simulink model "gap_generation_platoon"  (R2019a)
settings: Solver=VariableStepAuto  StartTime=0.0  StopTime=25  RelTol=1e-3
values from neighbouring files (symbols this model uses):
  ehMax = 3    [sim_parameters.m]
  ehMin = -100    [sim_parameters.m]
  g0 = 1/2*maxAccel*T^2 + maxAccel*T*t1 + + 1/2*maxAccel*t1^2 + 1/6*minJerk*t1^3 -      1/(2*minAccel)*(maxAccel*T + maxAccel*t1+ 1/2*minJerk*t1^2)^2    [safeHeadway.m]    (also in sim_parameters.m = ceil(g0*10)*1.1/10)
  h = figure()    [plotKinematicsFromSimulink.m]    (also in safeHeadway.m = T + t1 -      1/minAccel*(maxAccel*T + maxAccel*t1+1/2*minJe; sim_parameters.m = ceil(h*10)*1.1/10)
  Kd = K(1)    [SimulinkScenario.m]
  Ki = K(3)    [SimulinkScenario.m]
  Kp = K(2)    [SimulinkScenario.m]
  lcStartTime = 5    [SimulinkScenario.m]
  maxAcc = 4    [sim_parameters.m]
  maxJerk = 40    [sim_parameters.m]
  minAcc = -8    [sim_parameters.m]
  minJerk = -75    [sim_parameters.m]
  p = 10    [sim_parameters.m]
  vehMass = 2000    [sim_parameters.m]
  velKi = KiVelControl    [SimulinkScenario.m]
  vLen = lf+lr    (= 3)    [sim_parameters.m]
libraries: autolibshared x5
settings Model: Creator=fvall  LastModifiedBy=fvall

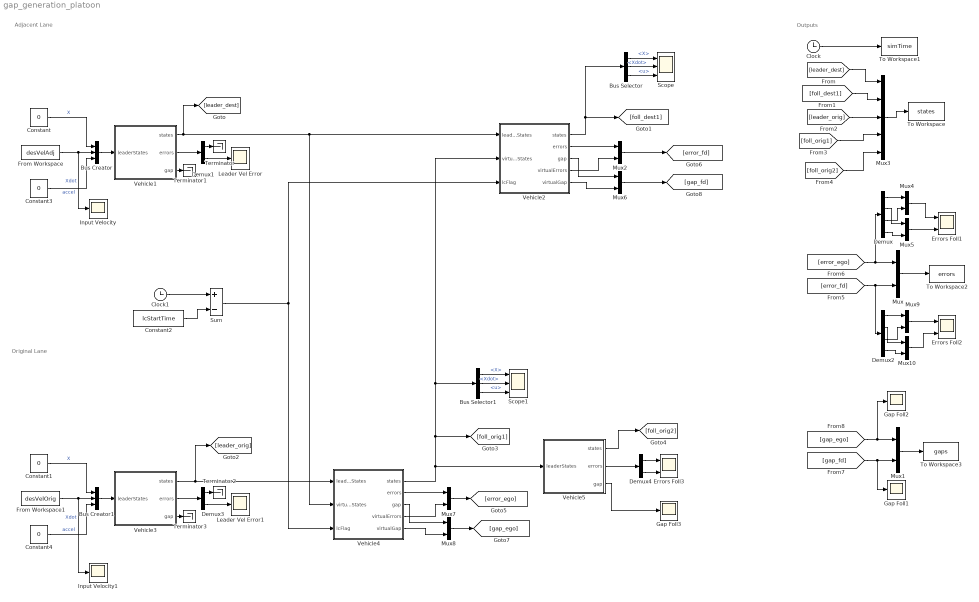
== system gap_generation_platoon ==
  note: Original Lane
  note: Adjacent Lane
  note: Outputs
  Bus Creator : BusCreator  Inputs=3
  Bus Creator1 : BusCreator  Inputs=3
  Bus Selector : BusSelector  OutputSignals=X,Xdot,u
  Bus Selector1 : BusSelector  OutputSignals=X,Xdot,u
  Clock : Clock
  Clock1 : Clock
  Constant{,1,3..4} (4 alike) : Constant  Value=0
  Constant2 : Constant  Value=lcStartTime
  Demux : Demux
  Demux1 : Demux  Outputs=2
  Demux2 : Demux
  Demux3 : Demux  Outputs=2
  Demux4 : Demux  Outputs=2
  Errors Foll1 : Scope  NumInputPorts=2
  Errors Foll2 : Scope  NumInputPorts=2
  Errors Foll3 : Scope  NumInputPorts=2
  From Workspace : FromWorkspace  VariableName=desVelAdj  SampleTime=0
  From Workspace1 : FromWorkspace  VariableName=desVelOrig  SampleTime=0
  Gap Foll1 : Scope
  Gap Foll2 : Scope
  Gap Foll3 : Scope
  Input Velocity : Scope
  Input Velocity1 : Scope
  Leader Vel Error : Scope
  Leader Vel Error1 : Scope
  Mux{,1..2,4..10} (10 alike) : Mux  Inputs=2
  Mux3 : Mux  Inputs=5
  Scope : Scope  NumInputPorts=3
  Scope1 : Scope  NumInputPorts=3
  Sum : Sum  Inputs=+-
  Terminator{,1..3} (4 alike) : Terminator
  To Workspace : ToWorkspace  VariableName=states  SampleTime=-1
  To Workspace1 : ToWorkspace  VariableName=simTime  SampleTime=-1
  To Workspace2 : ToWorkspace  VariableName=errors  SampleTime=-1
  To Workspace3 : ToWorkspace  VariableName=gaps  SampleTime=-1
  Vehicle1 : Subsystem  mask{m=vehMass, lf=vLen/2, lr=vLen/2, maxAcceleration=maxAcc, minAcceleration=minAcc, maxJerk=maxJerk, minJerk=minJerk, X_o=9.71, initVel=20, Y_o=3.6, h=h, g0=g0, minHeadwayError=ehMin, maxHeadwayError=ehMax, velFilterGain=p, Kd=Kd, Kp=Kp, Ki=Ki, VelKi=velKi}
      mask prompts: m "autoblks_shared:autoblkVehBody3DofLat:blkPrm_m"; lf "autoblks_shared:autoblkVehBody3DofLat:blkPrm_a"; lr "autoblks_shared:autoblkVehBody3DofLat:blkPrm_b"; maxAcceleration "Max Acceleration"; minAcceleration "Min Acceleration"; maxJerk "Max Jerk"; minJerk "Min Jerk"; X_o "autoblks_shared:autoblkVehBody3DofLat:blkPrm_X_o"; initVel "autoblks_shared:autoblkVehBody3DofLat:blkPrm_xdot_o"; Y_o "autoblks_shared:autoblkVehBody3DofLat:blkPrm_Y_o"; h "Time Headway"; g0 "Standstill Gap"; minHeadwayError "Min Headway Error"; maxHeadwayError "Max Headway Error"; velFilterGain "Velocity Filter Gain"
      mask TypeOptions m: Vehicle Body 3DOF Single Track/m
      mask TypeOptions lf: Vehicle Body 3DOF Single Track/a
      mask TypeOptions lr: Vehicle Body 3DOF Single Track/b
      mask TypeOptions X_o: Vehicle Body 3DOF Single Track/X_o
      mask TypeOptions initVel: Vehicle Body 3DOF Single Track/xdot_o
      mask TypeOptions Y_o: Vehicle Body 3DOF Single Track/Y_o
      mask TypeOptions Kd: ACC/Kd/Gain
      mask TypeOptions Kp: ACC/Kp/Gain
      mask TypeOptions Ki: ACC/Ki/Gain
      mask TypeOptions VelKi: ACC/VelKi/Gain
      mask DialogControl DescGroupVar Prompt: 3DOF Vehicle with ACC
      mask DialogControl DescTextVar Prompt: Vehicle with ACC. The vehicle model is Simulink's 3DOF single track vehicle body. The controller is a PID with constant headway including headway error saturation and filtered leader velocity.
      mask DialogControl ParameterGroupVar Prompt: Vehicle Parameters
      mask DialogControl m Prompt: Vehicle mass, m [kg]:
      mask DialogControl lf Prompt: Longitudinal distance from center of mass to front axle, a [m]:
      mask DialogControl lr Prompt: Longitudinal distance from center of mass to rear axle, b [m]:
      mask DialogControl X_o Prompt: Initial inertial frame longitudinal position, X_o [m]:
      mask DialogControl initVel Prompt: Initial longitudinal velocity, xdot_o [m/s]:
      mask DialogControl Y_o Prompt: Initial inertial frame lateral displacement, Y_o [m]:
      mask DialogControl Container3 Prompt: Controller Parameters
  Vehicle2 : Subsystem  mask{m=vehMass, lf=vLen/2, lr=vLen/2, maxAcceleration=maxAcc, minAcceleration=minAcc, maxJerk=maxJerk, minJerk=minJerk, X_o=0, initVel=20, Y_o=3.6, h=h, g0=g0, minHeadwayError=ehMin, maxHeadwayError=ehMax, velFilterGain=p, Kd=Kd, Kp=Kp, Ki=Ki, VelKi=velKi}
      mask prompts: m "autoblks_shared:autoblkVehBody3DofLat:blkPrm_m"; lf "autoblks_shared:autoblkVehBody3DofLat:blkPrm_a"; lr "autoblks_shared:autoblkVehBody3DofLat:blkPrm_b"; maxAcceleration "Max Acceleration"; minAcceleration "Min Acceleration"; maxJerk "Max Jerk"; minJerk "Min Jerk"; X_o "autoblks_shared:autoblkVehBody3DofLat:blkPrm_X_o"; initVel "autoblks_shared:autoblkVehBody3DofLat:blkPrm_xdot_o"; Y_o "autoblks_shared:autoblkVehBody3DofLat:blkPrm_Y_o"; h "Time Headway"; g0 "Standstill Gap"; minHeadwayError "Min Headway Error"; maxHeadwayError "Max Headway Error"; velFilterGain "Velocity Filter Gain"
      mask TypeOptions m: Vehicle Body 3DOF Single Track/m
      mask TypeOptions lf: Vehicle Body 3DOF Single Track/a
      mask TypeOptions lr: Vehicle Body 3DOF Single Track/b
      mask TypeOptions X_o: Vehicle Body 3DOF Single Track/X_o
      mask TypeOptions initVel: Vehicle Body 3DOF Single Track/xdot_o
      mask TypeOptions Y_o: Vehicle Body 3DOF Single Track/Y_o
      mask TypeOptions Kd: ACC/Kd/Gain
      mask TypeOptions Kp: ACC/Kp/Gain
      mask TypeOptions Ki: ACC/Ki/Gain
      mask TypeOptions VelKi: ACC/VelKi/Gain
      mask DialogControl DescGroupVar Prompt: 3DOF Vehicle with ACC
      mask DialogControl DescTextVar Prompt: Vehicle with ACC. The vehicle model is Simulink's 3DOF single track vehicle body. The controller is a PID with constant headway including headway error saturation and filtered leader velocity.
      mask DialogControl ParameterGroupVar Prompt: Vehicle Parameters
      mask DialogControl m Prompt: Vehicle mass, m [kg]:
      mask DialogControl lf Prompt: Longitudinal distance from center of mass to front axle, a [m]:
      mask DialogControl lr Prompt: Longitudinal distance from center of mass to rear axle, b [m]:
      mask DialogControl X_o Prompt: Initial inertial frame longitudinal position, X_o [m]:
      mask DialogControl initVel Prompt: Initial longitudinal velocity, xdot_o [m/s]:
      mask DialogControl Y_o Prompt: Initial inertial frame lateral displacement, Y_o [m]:
      mask DialogControl Container3 Prompt: Controller Parameters
  Vehicle3 : Subsystem  mask{m=vehMass, lf=vLen/2, lr=vLen/2, maxAcceleration=maxAcc, minAcceleration=minAcc, maxJerk=maxJerk, minJerk=minJerk, X_o=19.42, initVel=20, Y_o=0, h=h, g0=g0, minHeadwayError=ehMin, maxHeadwayError=ehMax, velFilterGain=p, Kd=Kd, Kp=Kp, Ki=Ki, VelKi=velKi}
      mask prompts: m "autoblks_shared:autoblkVehBody3DofLat:blkPrm_m"; lf "autoblks_shared:autoblkVehBody3DofLat:blkPrm_a"; lr "autoblks_shared:autoblkVehBody3DofLat:blkPrm_b"; maxAcceleration "Max Acceleration"; minAcceleration "Min Acceleration"; maxJerk "Max Jerk"; minJerk "Min Jerk"; X_o "autoblks_shared:autoblkVehBody3DofLat:blkPrm_X_o"; initVel "autoblks_shared:autoblkVehBody3DofLat:blkPrm_xdot_o"; Y_o "autoblks_shared:autoblkVehBody3DofLat:blkPrm_Y_o"; h "Time Headway"; g0 "Standstill Gap"; minHeadwayError "Min Headway Error"; maxHeadwayError "Max Headway Error"; velFilterGain "Velocity Filter Gain"
      mask TypeOptions m: Vehicle Body 3DOF Single Track/m
      mask TypeOptions lf: Vehicle Body 3DOF Single Track/a
      mask TypeOptions lr: Vehicle Body 3DOF Single Track/b
      mask TypeOptions X_o: Vehicle Body 3DOF Single Track/X_o
      mask TypeOptions initVel: Vehicle Body 3DOF Single Track/xdot_o
      mask TypeOptions Y_o: Vehicle Body 3DOF Single Track/Y_o
      mask TypeOptions Kd: ACC/Kd/Gain
      mask TypeOptions Kp: ACC/Kp/Gain
      mask TypeOptions Ki: ACC/Ki/Gain
      mask TypeOptions VelKi: ACC/VelKi/Gain
      mask DialogControl DescGroupVar Prompt: 3DOF Vehicle with ACC
      mask DialogControl DescTextVar Prompt: Vehicle with ACC. The vehicle model is Simulink's 3DOF single track vehicle body. The controller is a PID with constant headway including headway error saturation and filtered leader velocity.
      mask DialogControl ParameterGroupVar Prompt: Vehicle Parameters
      mask DialogControl m Prompt: Vehicle mass, m [kg]:
      mask DialogControl lf Prompt: Longitudinal distance from center of mass to front axle, a [m]:
      mask DialogControl lr Prompt: Longitudinal distance from center of mass to rear axle, b [m]:
      mask DialogControl X_o Prompt: Initial inertial frame longitudinal position, X_o [m]:
      mask DialogControl initVel Prompt: Initial longitudinal velocity, xdot_o [m/s]:
      mask DialogControl Y_o Prompt: Initial inertial frame lateral displacement, Y_o [m]:
      mask DialogControl Container3 Prompt: Controller Parameters
  Vehicle4 : Subsystem  mask{m=vehMass, lf=vLen/2, lr=vLen/2, maxAcceleration=maxAcc, minAcceleration=minAcc, maxJerk=maxJerk, minJerk=minJerk, X_o=9.71, initVel=20, Y_o=0, h=h, g0=g0, minHeadwayError=ehMin, maxHeadwayError=ehMax, velFilterGain=p, Kd=Kd, Kp=Kp, Ki=Ki, VelKi=velKi}
      mask prompts: m "autoblks_shared:autoblkVehBody3DofLat:blkPrm_m"; lf "autoblks_shared:autoblkVehBody3DofLat:blkPrm_a"; lr "autoblks_shared:autoblkVehBody3DofLat:blkPrm_b"; maxAcceleration "Max Acceleration"; minAcceleration "Min Acceleration"; maxJerk "Max Jerk"; minJerk "Min Jerk"; X_o "autoblks_shared:autoblkVehBody3DofLat:blkPrm_X_o"; initVel "autoblks_shared:autoblkVehBody3DofLat:blkPrm_xdot_o"; Y_o "autoblks_shared:autoblkVehBody3DofLat:blkPrm_Y_o"; h "Time Headway"; g0 "Standstill Gap"; minHeadwayError "Min Headway Error"; maxHeadwayError "Max Headway Error"; velFilterGain "Velocity Filter Gain"
      mask TypeOptions m: Vehicle Body 3DOF Single Track/m
      mask TypeOptions lf: Vehicle Body 3DOF Single Track/a
      mask TypeOptions lr: Vehicle Body 3DOF Single Track/b
      mask TypeOptions X_o: Vehicle Body 3DOF Single Track/X_o
      mask TypeOptions initVel: Vehicle Body 3DOF Single Track/xdot_o
      mask TypeOptions Y_o: Vehicle Body 3DOF Single Track/Y_o
      mask TypeOptions Kd: ACC/Kd/Gain
      mask TypeOptions Kp: ACC/Kp/Gain
      mask TypeOptions Ki: ACC/Ki/Gain
      mask TypeOptions VelKi: ACC/VelKi/Gain
      mask DialogControl DescGroupVar Prompt: 3DOF Vehicle with ACC
      mask DialogControl DescTextVar Prompt: Vehicle with ACC. The vehicle model is Simulink's 3DOF single track vehicle body. The controller is a PID with constant headway including headway error saturation and filtered leader velocity.
      mask DialogControl ParameterGroupVar Prompt: Vehicle Parameters
      mask DialogControl m Prompt: Vehicle mass, m [kg]:
      mask DialogControl lf Prompt: Longitudinal distance from center of mass to front axle, a [m]:
      mask DialogControl lr Prompt: Longitudinal distance from center of mass to rear axle, b [m]:
      mask DialogControl X_o Prompt: Initial inertial frame longitudinal position, X_o [m]:
      mask DialogControl initVel Prompt: Initial longitudinal velocity, xdot_o [m/s]:
      mask DialogControl Y_o Prompt: Initial inertial frame lateral displacement, Y_o [m]:
      mask DialogControl Container3 Prompt: Controller Parameters
  Vehicle5 : Subsystem  mask{m=vehMass, lf=vLen/2, lr=vLen/2, maxAcceleration=maxAcc, minAcceleration=minAcc, maxJerk=maxJerk, minJerk=minJerk, X_o=0, initVel=20, Y_o=0, h=h, g0=g0, minHeadwayError=ehMin, maxHeadwayError=ehMax, velFilterGain=p, Kd=Kd, Kp=Kp, Ki=Ki, VelKi=velKi}
      mask prompts: m "autoblks_shared:autoblkVehBody3DofLat:blkPrm_m"; lf "autoblks_shared:autoblkVehBody3DofLat:blkPrm_a"; lr "autoblks_shared:autoblkVehBody3DofLat:blkPrm_b"; maxAcceleration "Max Acceleration"; minAcceleration "Min Acceleration"; maxJerk "Max Jerk"; minJerk "Min Jerk"; X_o "autoblks_shared:autoblkVehBody3DofLat:blkPrm_X_o"; initVel "autoblks_shared:autoblkVehBody3DofLat:blkPrm_xdot_o"; Y_o "autoblks_shared:autoblkVehBody3DofLat:blkPrm_Y_o"; h "Time Headway"; g0 "Standstill Gap"; minHeadwayError "Min Headway Error"; maxHeadwayError "Max Headway Error"; velFilterGain "Velocity Filter Gain"
      mask TypeOptions m: Vehicle Body 3DOF Single Track/m
      mask TypeOptions lf: Vehicle Body 3DOF Single Track/a
      mask TypeOptions lr: Vehicle Body 3DOF Single Track/b
      mask TypeOptions X_o: Vehicle Body 3DOF Single Track/X_o
      mask TypeOptions initVel: Vehicle Body 3DOF Single Track/xdot_o
      mask TypeOptions Y_o: Vehicle Body 3DOF Single Track/Y_o
      mask TypeOptions Kd: ACC/Kd/Gain
      mask TypeOptions Kp: ACC/Kp/Gain
      mask TypeOptions Ki: ACC/Ki/Gain
      mask TypeOptions VelKi: ACC/VelKi/Gain
      mask DialogControl DescGroupVar Prompt: 3DOF Vehicle with ACC
      mask DialogControl DescTextVar Prompt: Vehicle with ACC. The vehicle model is Simulink's 3DOF single track vehicle body. The controller is a PID with constant headway including headway error saturation and filtered leader velocity.
      mask DialogControl ParameterGroupVar Prompt: Vehicle Parameters
      mask DialogControl m Prompt: Vehicle mass, m [kg]:
      mask DialogControl lf Prompt: Longitudinal distance from center of mass to front axle, a [m]:
      mask DialogControl lr Prompt: Longitudinal distance from center of mass to rear axle, b [m]:
      mask DialogControl X_o Prompt: Initial inertial frame longitudinal position, X_o [m]:
      mask DialogControl initVel Prompt: Initial longitudinal velocity, xdot_o [m/s]:
      mask DialogControl Y_o Prompt: Initial inertial frame lateral displacement, Y_o [m]:
      mask DialogControl Container3 Prompt: Controller Parameters
  wires:
  Vehicle2/1(states) -> Bus Selector/1, [foll_dest1]
  Demux1/1 -> Terminator/1
  Demux1/2 -> Leader Vel Error/1
  Vehicle1/3(gap) -> Terminator1/1
  From Workspace/1 -> Bus Creator/2, Input Velocity/1  "Xdot"
  Vehicle1/2(errors) -> Demux1/1
  Clock/1 -> To Workspace1/1
  [foll_dest1] -> Mux3/2
  [leader_dest] -> Mux3/1
  Mux3/1 -> To Workspace/1
  Demux3/2 -> Leader Vel Error1/1
  Demux3/1 -> Terminator2/1
  Vehicle4/1(states) -> Vehicle5/1(leaderStates), Bus Selector1/1, Vehicle2/2(virtualLeaderStates), [foll_orig1]
  Vehicle3/1(states) -> [leader_orig], Vehicle4/1(leaderStates)
  Vehicle3/3(gap) -> Terminator3/1
  [leader_orig] -> Mux3/3
  [foll_orig1] -> Mux3/4
  Vehicle5/3(gap) -> Gap Foll3/1
  Vehicle5/2(errors) -> Demux4/1
  Demux4/1 -> Errors Foll3/1
  Demux4/2 -> Errors Foll3/2
  [foll_orig2] -> Mux3/5
  Constant/1 -> Bus Creator/1  "X"
  Constant3/1 -> Bus Creator/3  "accel"
  Bus Creator/1 -> Vehicle1/1(leaderStates)
  Vehicle1/1(states) -> Vehicle2/1(leaderStates), Vehicle4/2(virtualLeaderStates), [leader_dest]
  Constant4/1 -> Bus Creator1/3  "accel"
  From Workspace1/1 -> Bus Creator1/2, Input Velocity1/1  "Xdot"
  Constant1/1 -> Bus Creator1/1  "X"
  Bus Creator1/1 -> Vehicle3/1(leaderStates)
  Vehicle3/2(errors) -> Demux3/1
  Clock1/1 -> Sum/1
  Constant2/1 -> Sum/2
  Mux/1 -> To Workspace2/1
  [gap_ego] -> Gap Foll2/1, Mux1/1
  [gap_fd] -> Gap Foll1/1, Mux1/2
  Mux1/1 -> To Workspace3/1
  Sum/1 -> Vehicle2/3(lcFlag), Vehicle4/3(lcFlag)
  Vehicle2/2(errors) -> Mux2/1
  Vehicle2/4(virtualErrors) -> Mux2/2
  Mux2/1 -> [error_fd]
  Vehicle2/3(gap) -> Mux6/1
  Vehicle2/5(virtualGap) -> Mux6/2
  Mux6/1 -> [gap_fd]
  Vehicle4/3(gap) -> Mux8/1
  Vehicle4/5(virtualGap) -> Mux8/2
  Vehicle4/2(errors) -> Mux7/1
  Vehicle4/4(virtualErrors) -> Mux7/2
  Mux7/1 -> [error_ego]
  Mux8/1 -> [gap_ego]
  Demux/3 -> Mux4/2
  Mux5/1 -> Errors Foll1/2
  Demux/1 -> Mux4/1
  Demux/2 -> Mux5/1
  Demux/4 -> Mux5/2
  [error_ego] -> Demux/1, Mux/1
  Mux4/1 -> Errors Foll1/1
  Demux2/1 -> Mux9/1
  Mux9/1 -> Errors Foll2/1
  Demux2/4 -> Mux10/2
  Mux10/1 -> Errors Foll2/2
  Demux2/2 -> Mux10/1
  Demux2/3 -> Mux9/2
  [error_fd] -> Demux2/1, Mux/2
  Bus Selector/1 -> Scope/1  "<X>"
  Bus Selector/2 -> Scope/2  "<Xdot>"
  Vehicle5/1(states) -> [foll_orig2]
  Bus Selector/3 -> Scope/3  "<u>"
  Bus Selector1/1 -> Scope1/1  "<X>"
  Bus Selector1/2 -> Scope1/2  "<Xdot>"
  Bus Selector1/3 -> Scope1/3  "<u>"

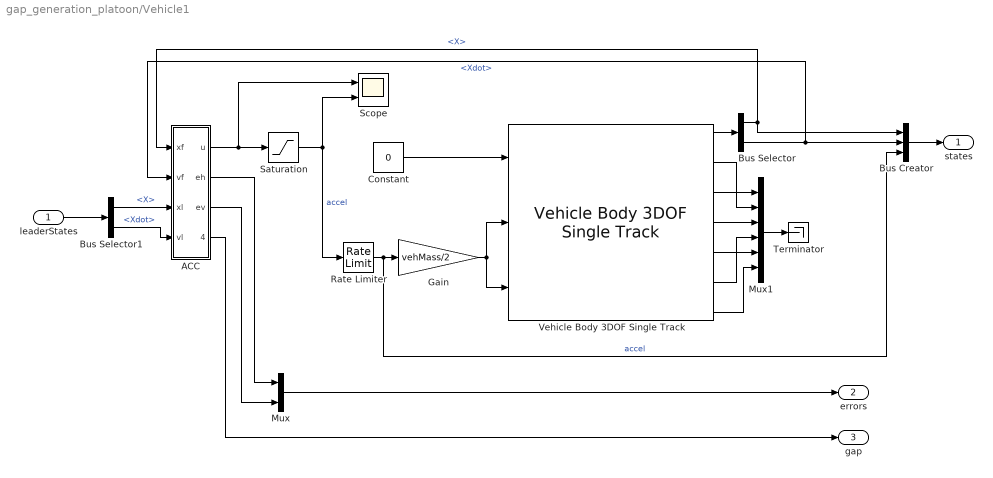
== system gap_generation_platoon/Vehicle1 ==
  leaderStates : Inport
  ACC : Subsystem
  Bus Creator : BusCreator  Inputs=3
  Bus Selector : BusSelector  OutputSignals=InertFrm.RearAxl.Disp.X,InertFrm.RearAxl.Vel.Xdot
  Bus Selector1 : BusSelector  OutputSignals=X,Xdot
  Constant : Constant  Value=0
  Gain : Gain  Gain=vehMass/2
  Mux : Mux  Inputs=2
  Mux1 : Mux  Inputs=6
  Rate Limiter : RateLimiter  RisingSlewLimit=maxJerk  FallingSlewLimit=minJerk  SampleTimeMode=inherited
  Saturation : Saturate  UpperLimit=maxAcc  LowerLimit=minAcc
  Scope : Scope  NumInputPorts=2
  Terminator : Terminator
  Vehicle Body 3DOF Single Track : autolibshared/Vehicle Body 3DOF Single Track  trackMode=Single (bicycle)  inputMode=External longitudinal forces  frontSteerMode=on  rearSteerMode=off  windMode=off  muMode=off  extFMode=off  extMMode=off  extXo=off  extpsio=off  extxdoto=off  extro=off  extYo=off  extTamb=off  extydoto=off  aMode=2  NF=2  NR=2  m=m  a=lf  b=lr  h=0.35  X_o=X_o  xdot_o=initVel  CalphaMode=off  sigmaMode=on  d=0  w=[1.4,1.4]  Cy_f=12e3  Cy_r=11e3  sigma_f=.1  sigma_r=.1  alpha_f_brk=[-.1 .1]  Cy_f_data=[-9e3 9e3]  alpha_r_brk=[-.1 .1]  Cy_r_data=[-9e3 9e3]  Y_o=Y_o  ydot_o=0  Izz=4000  psi_o=0  r_o=0  Af=2  Cd=.3  Cl=.1  Cpm=.1  beta_w=[0:0.01:0.3]  Cs=[0:0.03:0.9]  Cym=[0:0.01:0.3]  Pabs=101325  Tair=273  g=9.81  mu=1  xdot_tol=.01  Fznom=5000  Fxtire_sat=7e4  Fytire_sat=7e4  longOff=0  latOff=0  vertOff=0  wrapAng=off
      settings: SourceProductName=Powertrain Blockset  SourceProductBaseCode=PW
  states : Outport
  errors : Outport  Port=2
  gap : Outport  Port=3
  wires:
  Bus Selector/2 -> Bus Creator/2, ACC/2(vf)  "<Xdot>"
  Bus Selector/1 -> Bus Creator/1, ACC/1(xf)  "<X>"
  Saturation/1 -> Scope/2, Rate Limiter/1  "accel"
  ACC/1(u) -> Scope/1, Saturation/1
  ACC/2(eh) -> Mux/1
  ACC/3(ev) -> Mux/2
  Mux/1 -> errors/1
  Gain/1 -> Vehicle Body 3DOF Single Track/2, Vehicle Body 3DOF Single Track/3
  Constant/1 -> Vehicle Body 3DOF Single Track/1
  Vehicle Body 3DOF Single Track/1 -> Bus Selector/1
  Vehicle Body 3DOF Single Track/4 -> Mux1/3
  Vehicle Body 3DOF Single Track/3 -> Mux1/2
  Vehicle Body 3DOF Single Track/2 -> Mux1/1
  Vehicle Body 3DOF Single Track/5 -> Mux1/4
  Vehicle Body 3DOF Single Track/6 -> Mux1/5
  Vehicle Body 3DOF Single Track/7 -> Mux1/6
  Mux1/1 -> Terminator/1
  ACC/4(gap) -> gap/1
  Rate Limiter/1 -> Bus Creator/3, Gain/1  "accel"
  Bus Creator/1 -> states/1
  leaderStates/1 -> Bus Selector1/1
  Bus Selector1/1 -> ACC/3(xl)  "<X>"
  Bus Selector1/2 -> ACC/4(vl)  "<Xdot>"

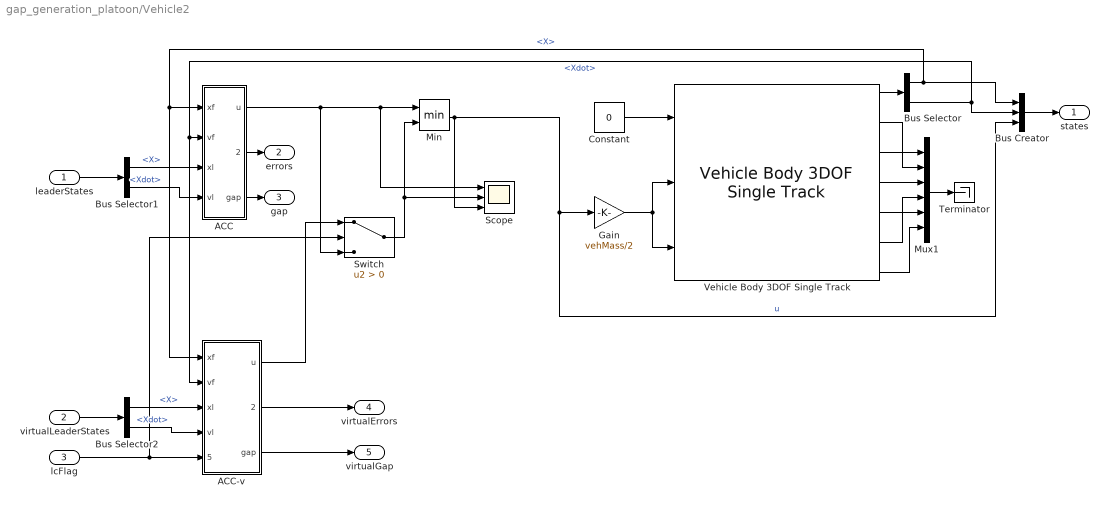
== system gap_generation_platoon/Vehicle2 ==
  leaderStates : Inport
  virtualLeaderStates : Inport  Port=2
  lcFlag : Inport  Port=3
  ACC : Subsystem
  ACC-v : Subsystem
  Bus Creator : BusCreator  Inputs=3
  Bus Selector : BusSelector  OutputSignals=InertFrm.RearAxl.Disp.X,InertFrm.RearAxl.Vel.Xdot
  Bus Selector1 : BusSelector  OutputSignals=X,Xdot
  Bus Selector2 : BusSelector  OutputSignals=X,Xdot
  Constant : Constant  Value=0
  Gain : Gain  Gain=vehMass/2
  Min : MinMax  Inputs=2
  Mux1 : Mux  Inputs=6
  Scope : Scope  NumInputPorts=3
  Switch : Switch  Criteria=u2 > Threshold
  Terminator : Terminator
  Vehicle Body 3DOF Single Track : autolibshared/Vehicle Body 3DOF Single Track  trackMode=Single (bicycle)  inputMode=External longitudinal forces  frontSteerMode=on  rearSteerMode=off  windMode=off  muMode=off  extFMode=off  extMMode=off  extXo=off  extpsio=off  extxdoto=off  extro=off  extYo=off  extTamb=off  extydoto=off  aMode=2  NF=2  NR=2  m=m  a=lf  b=lr  h=0.35  X_o=X_o  xdot_o=initVel  CalphaMode=off  sigmaMode=on  d=0  w=[1.4,1.4]  Cy_f=12e3  Cy_r=11e3  sigma_f=.1  sigma_r=.1  alpha_f_brk=[-.1 .1]  Cy_f_data=[-9e3 9e3]  alpha_r_brk=[-.1 .1]  Cy_r_data=[-9e3 9e3]  Y_o=Y_o  ydot_o=0  Izz=4000  psi_o=0  r_o=0  Af=2  Cd=.3  Cl=.1  Cpm=.1  beta_w=[0:0.01:0.3]  Cs=[0:0.03:0.9]  Cym=[0:0.01:0.3]  Pabs=101325  Tair=273  g=9.81  mu=1  xdot_tol=.01  Fznom=5000  Fxtire_sat=7e4  Fytire_sat=7e4  longOff=0  latOff=0  vertOff=0  wrapAng=off
      settings: SourceProductName=Powertrain Blockset  SourceProductBaseCode=PW
  states : Outport
  errors : Outport  Port=2
  gap : Outport  Port=3
  virtualErrors : Outport  Port=4
  virtualGap : Outport  Port=5
  wires:
  Bus Selector/2 -> Bus Creator/2, ACC-v/2(vf), ACC/2(vf)  "<Xdot>"
  Bus Selector/1 -> Bus Creator/1, ACC-v/1(xf), ACC/1(xf)  "<X>"
  Min/1 -> Bus Creator/3, Gain/1, Scope/3  "u"
  ACC/1(u) -> Switch/3, Min/1, Scope/1
  Gain/1 -> Vehicle Body 3DOF Single Track/3, Vehicle Body 3DOF Single Track/2
  Constant/1 -> Vehicle Body 3DOF Single Track/1
  Vehicle Body 3DOF Single Track/1 -> Bus Selector/1
  Vehicle Body 3DOF Single Track/4 -> Mux1/3
  Vehicle Body 3DOF Single Track/3 -> Mux1/2
  Vehicle Body 3DOF Single Track/2 -> Mux1/1
  Vehicle Body 3DOF Single Track/5 -> Mux1/4
  Vehicle Body 3DOF Single Track/6 -> Mux1/5
  Vehicle Body 3DOF Single Track/7 -> Mux1/6
  Mux1/1 -> Terminator/1
  ACC/3(gap) -> gap/1
  Bus Creator/1 -> states/1
  leaderStates/1 -> Bus Selector1/1
  Bus Selector1/1 -> ACC/3(xl)  "<X>"
  Bus Selector1/2 -> ACC/4(vl)  "<Xdot>"
  Bus Selector2/1 -> ACC-v/3(xl)  "<X>"
  Bus Selector2/2 -> ACC-v/4(vl)  "<Xdot>"
  ACC/2(errors) -> errors/1
  lcFlag/1 -> Switch/2, ACC-v/5(lcFlag)
  Switch/1 -> Min/2, Scope/2
  virtualLeaderStates/1 -> Bus Selector2/1
  ACC-v/1(u) -> Switch/1
  ACC-v/2(errors) -> virtualErrors/1
  ACC-v/3(gap) -> virtualGap/1

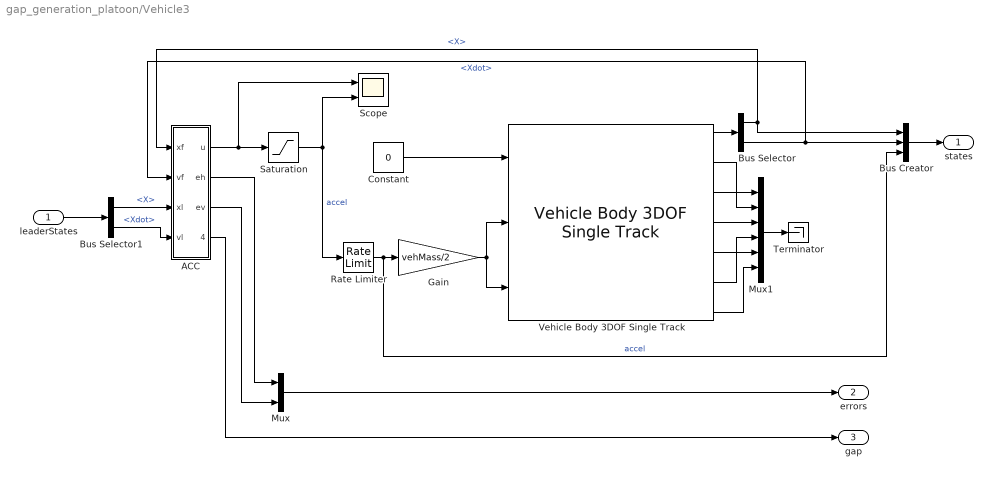
== system gap_generation_platoon/Vehicle3 ==
  leaderStates : Inport
  ACC : Subsystem
  Bus Creator : BusCreator  Inputs=3
  Bus Selector : BusSelector  OutputSignals=InertFrm.RearAxl.Disp.X,InertFrm.RearAxl.Vel.Xdot
  Bus Selector1 : BusSelector  OutputSignals=X,Xdot
  Constant : Constant  Value=0
  Gain : Gain  Gain=vehMass/2
  Mux : Mux  Inputs=2
  Mux1 : Mux  Inputs=6
  Rate Limiter : RateLimiter  RisingSlewLimit=maxJerk  FallingSlewLimit=minJerk  SampleTimeMode=inherited
  Saturation : Saturate  UpperLimit=maxAcc  LowerLimit=minAcc
  Scope : Scope  NumInputPorts=2
  Terminator : Terminator
  Vehicle Body 3DOF Single Track : autolibshared/Vehicle Body 3DOF Single Track  trackMode=Single (bicycle)  inputMode=External longitudinal forces  frontSteerMode=on  rearSteerMode=off  windMode=off  muMode=off  extFMode=off  extMMode=off  extXo=off  extpsio=off  extxdoto=off  extro=off  extYo=off  extTamb=off  extydoto=off  aMode=2  NF=2  NR=2  m=m  a=lf  b=lr  h=0.35  X_o=X_o  xdot_o=initVel  CalphaMode=off  sigmaMode=on  d=0  w=[1.4,1.4]  Cy_f=12e3  Cy_r=11e3  sigma_f=.1  sigma_r=.1  alpha_f_brk=[-.1 .1]  Cy_f_data=[-9e3 9e3]  alpha_r_brk=[-.1 .1]  Cy_r_data=[-9e3 9e3]  Y_o=Y_o  ydot_o=0  Izz=4000  psi_o=0  r_o=0  Af=2  Cd=.3  Cl=.1  Cpm=.1  beta_w=[0:0.01:0.3]  Cs=[0:0.03:0.9]  Cym=[0:0.01:0.3]  Pabs=101325  Tair=273  g=9.81  mu=1  xdot_tol=.01  Fznom=5000  Fxtire_sat=7e4  Fytire_sat=7e4  longOff=0  latOff=0  vertOff=0  wrapAng=off
      settings: SourceProductName=Powertrain Blockset  SourceProductBaseCode=PW
  states : Outport
  errors : Outport  Port=2
  gap : Outport  Port=3
  wires:
  Bus Selector/2 -> Bus Creator/2, ACC/2(vf)  "<Xdot>"
  Bus Selector/1 -> Bus Creator/1, ACC/1(xf)  "<X>"
  Saturation/1 -> Scope/2, Rate Limiter/1  "accel"
  ACC/1(u) -> Scope/1, Saturation/1
  ACC/2(eh) -> Mux/1
  ACC/3(ev) -> Mux/2
  Mux/1 -> errors/1
  Gain/1 -> Vehicle Body 3DOF Single Track/2, Vehicle Body 3DOF Single Track/3
  Constant/1 -> Vehicle Body 3DOF Single Track/1
  Vehicle Body 3DOF Single Track/1 -> Bus Selector/1
  Vehicle Body 3DOF Single Track/4 -> Mux1/3
  Vehicle Body 3DOF Single Track/3 -> Mux1/2
  Vehicle Body 3DOF Single Track/2 -> Mux1/1
  Vehicle Body 3DOF Single Track/5 -> Mux1/4
  Vehicle Body 3DOF Single Track/6 -> Mux1/5
  Vehicle Body 3DOF Single Track/7 -> Mux1/6
  Mux1/1 -> Terminator/1
  ACC/4(gap) -> gap/1
  Rate Limiter/1 -> Bus Creator/3, Gain/1  "accel"
  Bus Creator/1 -> states/1
  leaderStates/1 -> Bus Selector1/1
  Bus Selector1/1 -> ACC/3(xl)  "<X>"
  Bus Selector1/2 -> ACC/4(vl)  "<Xdot>"

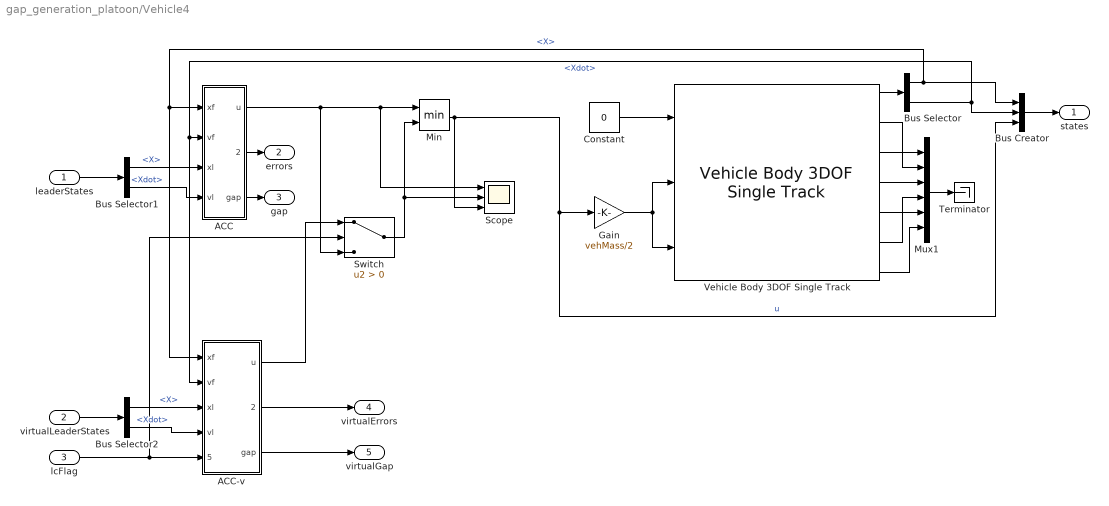
== system gap_generation_platoon/Vehicle4 ==
  leaderStates : Inport
  virtualLeaderStates : Inport  Port=2
  lcFlag : Inport  Port=3
  ACC : Subsystem
  ACC-v : Subsystem
  Bus Creator : BusCreator  Inputs=3
  Bus Selector : BusSelector  OutputSignals=InertFrm.RearAxl.Disp.X,InertFrm.RearAxl.Vel.Xdot
  Bus Selector1 : BusSelector  OutputSignals=X,Xdot
  Bus Selector2 : BusSelector  OutputSignals=X,Xdot
  Constant : Constant  Value=0
  Gain : Gain  Gain=vehMass/2
  Min : MinMax  Inputs=2
  Mux1 : Mux  Inputs=6
  Scope : Scope  NumInputPorts=3
  Switch : Switch  Criteria=u2 > Threshold
  Terminator : Terminator
  Vehicle Body 3DOF Single Track : autolibshared/Vehicle Body 3DOF Single Track  trackMode=Single (bicycle)  inputMode=External longitudinal forces  frontSteerMode=on  rearSteerMode=off  windMode=off  muMode=off  extFMode=off  extMMode=off  extXo=off  extpsio=off  extxdoto=off  extro=off  extYo=off  extTamb=off  extydoto=off  aMode=2  NF=2  NR=2  m=m  a=lf  b=lr  h=0.35  X_o=X_o  xdot_o=initVel  CalphaMode=off  sigmaMode=on  d=0  w=[1.4,1.4]  Cy_f=12e3  Cy_r=11e3  sigma_f=.1  sigma_r=.1  alpha_f_brk=[-.1 .1]  Cy_f_data=[-9e3 9e3]  alpha_r_brk=[-.1 .1]  Cy_r_data=[-9e3 9e3]  Y_o=Y_o  ydot_o=0  Izz=4000  psi_o=0  r_o=0  Af=2  Cd=.3  Cl=.1  Cpm=.1  beta_w=[0:0.01:0.3]  Cs=[0:0.03:0.9]  Cym=[0:0.01:0.3]  Pabs=101325  Tair=273  g=9.81  mu=1  xdot_tol=.01  Fznom=5000  Fxtire_sat=7e4  Fytire_sat=7e4  longOff=0  latOff=0  vertOff=0  wrapAng=off
      settings: SourceProductName=Powertrain Blockset  SourceProductBaseCode=PW
  states : Outport
  errors : Outport  Port=2
  gap : Outport  Port=3
  virtualErrors : Outport  Port=4
  virtualGap : Outport  Port=5
  wires:
  Bus Selector/2 -> Bus Creator/2, ACC-v/2(vf), ACC/2(vf)  "<Xdot>"
  Bus Selector/1 -> Bus Creator/1, ACC-v/1(xf), ACC/1(xf)  "<X>"
  Min/1 -> Bus Creator/3, Gain/1, Scope/3  "u"
  ACC/1(u) -> Switch/3, Min/1, Scope/1
  Gain/1 -> Vehicle Body 3DOF Single Track/3, Vehicle Body 3DOF Single Track/2
  Constant/1 -> Vehicle Body 3DOF Single Track/1
  Vehicle Body 3DOF Single Track/1 -> Bus Selector/1
  Vehicle Body 3DOF Single Track/4 -> Mux1/3
  Vehicle Body 3DOF Single Track/3 -> Mux1/2
  Vehicle Body 3DOF Single Track/2 -> Mux1/1
  Vehicle Body 3DOF Single Track/5 -> Mux1/4
  Vehicle Body 3DOF Single Track/6 -> Mux1/5
  Vehicle Body 3DOF Single Track/7 -> Mux1/6
  Mux1/1 -> Terminator/1
  ACC/3(gap) -> gap/1
  Bus Creator/1 -> states/1
  leaderStates/1 -> Bus Selector1/1
  Bus Selector1/1 -> ACC/3(xl)  "<X>"
  Bus Selector1/2 -> ACC/4(vl)  "<Xdot>"
  Bus Selector2/1 -> ACC-v/3(xl)  "<X>"
  Bus Selector2/2 -> ACC-v/4(vl)  "<Xdot>"
  ACC/2(errors) -> errors/1
  lcFlag/1 -> Switch/2, ACC-v/5(lcFlag)
  Switch/1 -> Min/2, Scope/2
  virtualLeaderStates/1 -> Bus Selector2/1
  ACC-v/1(u) -> Switch/1
  ACC-v/2(errors) -> virtualErrors/1
  ACC-v/3(gap) -> virtualGap/1

== system gap_generation_platoon/Vehicle5 ==
  leaderStates : Inport
  ACC : Subsystem
  Bus Creator : BusCreator  Inputs=3
  Bus Selector : BusSelector  OutputSignals=InertFrm.RearAxl.Disp.X,InertFrm.RearAxl.Vel.Xdot
  Bus Selector1 : BusSelector  OutputSignals=X,Xdot
  Constant : Constant  Value=0
  Gain : Gain  Gain=vehMass/2
  Mux : Mux  Inputs=2
  Mux1 : Mux  Inputs=6
  Rate Limiter : RateLimiter  RisingSlewLimit=maxJerk  FallingSlewLimit=minJerk  SampleTimeMode=inherited
  Saturation : Saturate  UpperLimit=maxAcc  LowerLimit=minAcc
  Scope : Scope  NumInputPorts=2
  Terminator : Terminator
  Vehicle Body 3DOF Single Track : autolibshared/Vehicle Body 3DOF Single Track  trackMode=Single (bicycle)  inputMode=External longitudinal forces  frontSteerMode=on  rearSteerMode=off  windMode=off  muMode=off  extFMode=off  extMMode=off  extXo=off  extpsio=off  extxdoto=off  extro=off  extYo=off  extTamb=off  extydoto=off  aMode=2  NF=2  NR=2  m=m  a=lf  b=lr  h=0.35  X_o=X_o  xdot_o=initVel  CalphaMode=off  sigmaMode=on  d=0  w=[1.4,1.4]  Cy_f=12e3  Cy_r=11e3  sigma_f=.1  sigma_r=.1  alpha_f_brk=[-.1 .1]  Cy_f_data=[-9e3 9e3]  alpha_r_brk=[-.1 .1]  Cy_r_data=[-9e3 9e3]  Y_o=Y_o  ydot_o=0  Izz=4000  psi_o=0  r_o=0  Af=2  Cd=.3  Cl=.1  Cpm=.1  beta_w=[0:0.01:0.3]  Cs=[0:0.03:0.9]  Cym=[0:0.01:0.3]  Pabs=101325  Tair=273  g=9.81  mu=1  xdot_tol=.01  Fznom=5000  Fxtire_sat=7e4  Fytire_sat=7e4  longOff=0  latOff=0  vertOff=0  wrapAng=off
      settings: SourceProductName=Powertrain Blockset  SourceProductBaseCode=PW
  states : Outport
  errors : Outport  Port=2
  gap : Outport  Port=3
  wires:
  Bus Selector/2 -> Bus Creator/2, ACC/2(vf)  "<Xdot>"
  Bus Selector/1 -> Bus Creator/1, ACC/1(xf)  "<X>"
  Saturation/1 -> Scope/2, Rate Limiter/1  "accel"
  ACC/1(u) -> Scope/1, Saturation/1
  ACC/2(eh) -> Mux/1
  ACC/3(ev) -> Mux/2
  Mux/1 -> errors/1
  Gain/1 -> Vehicle Body 3DOF Single Track/2, Vehicle Body 3DOF Single Track/3
  Constant/1 -> Vehicle Body 3DOF Single Track/1
  Vehicle Body 3DOF Single Track/1 -> Bus Selector/1
  Vehicle Body 3DOF Single Track/4 -> Mux1/3
  Vehicle Body 3DOF Single Track/3 -> Mux1/2
  Vehicle Body 3DOF Single Track/2 -> Mux1/1
  Vehicle Body 3DOF Single Track/5 -> Mux1/4
  Vehicle Body 3DOF Single Track/6 -> Mux1/5
  Vehicle Body 3DOF Single Track/7 -> Mux1/6
  Mux1/1 -> Terminator/1
  ACC/4(gap) -> gap/1
  Rate Limiter/1 -> Bus Creator/3, Gain/1  "accel"
  Bus Creator/1 -> states/1
  leaderStates/1 -> Bus Selector1/1
  Bus Selector1/1 -> ACC/3(xl)  "<X>"
  Bus Selector1/2 -> ACC/4(vl)  "<Xdot>"

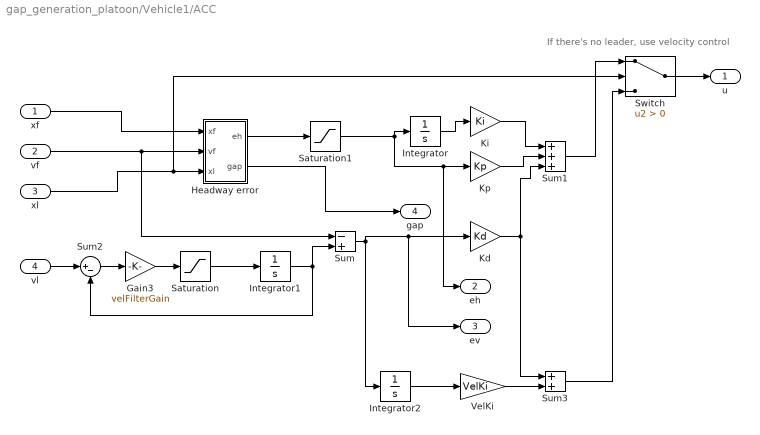
== system gap_generation_platoon/Vehicle1/ACC ==
  note: If there's no leader, use velocity control
  xf : Inport
  vf : Inport  Port=2
  xl : Inport  Port=3
  vl : Inport  Port=4
  Gain3 : Gain  Gain=velFilterGain
  Headway error : Subsystem  mask{vLen=vLen, g0=g0, h=h}
      mask prompts: vLen "Vehicle Length"; g0 "Standstill Gap"; h "Time Headway"
      mask init:
      | vLen >= 0;
      | g0 >= 0;
      | h >= 0;
  Integrator : Integrator
  Integrator1 : Integrator  InitialCondition=initVel
  Integrator2 : Integrator
  Kd : Gain  Gain=Kd
  Ki : Gain  Gain=Ki
  Kp : Gain  Gain=Kp
  Saturation : Saturate  UpperLimit=maxAcceleration  LowerLimit=minAcceleration
  Saturation1 : Saturate  UpperLimit=maxHeadwayError  LowerLimit=minHeadwayError
  Sum : Sum  Inputs=-+
  Sum1 : Sum  Inputs=+++
  Sum2 : Sum  Inputs=|+-
  Sum3 : Sum
  Switch : Switch  Criteria=u2 > Threshold
  VelKi : Gain  Gain=VelKi
  u : Outport
  eh : Outport  Port=2
  ev : Outport  Port=3
  gap : Outport  Port=4
  wires:
  Headway error/1(eh) -> Saturation1/1
  vf/1 -> Sum/1, Headway error/2(vf)
  Kd/1 -> Sum3/1, Sum1/3
  Kp/1 -> Sum1/2
  Ki/1 -> Sum1/1
  Integrator/1 -> Ki/1
  xl/1 -> Switch/2, Headway error/3(xl)
  xf/1 -> Headway error/1(xf)
  Gain3/1 -> Saturation/1
  Saturation/1 -> Integrator1/1
  Integrator1/1 -> Sum2/2, Sum/2
  vl/1 -> Sum2/1
  Sum2/1 -> Gain3/1
  Saturation1/1 -> eh/1, Kp/1, Integrator/1
  Headway error/2("gap ") -> gap/1
  Integrator2/1 -> VelKi/1
  VelKi/1 -> Sum3/2
  Switch/1 -> u/1
  Sum1/1 -> Switch/1
  Sum3/1 -> Switch/3
  Sum/1 -> ev/1, Kd/1, Integrator2/1

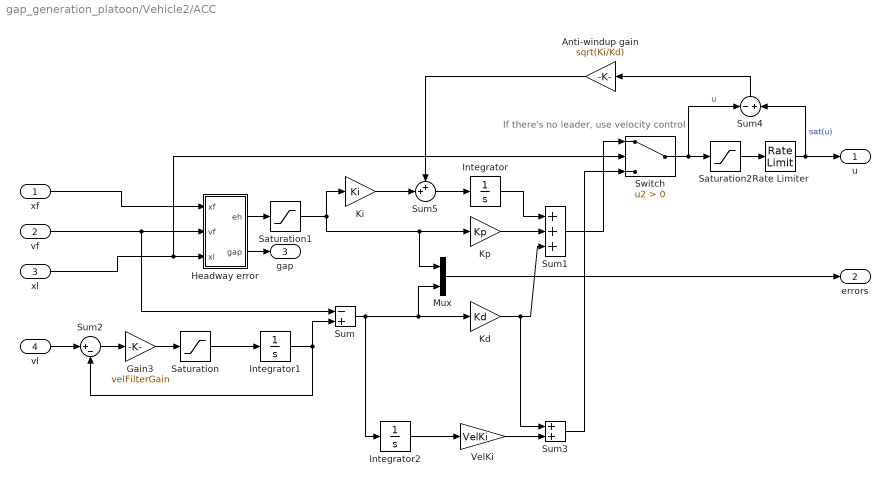
== system gap_generation_platoon/Vehicle2/ACC ==
  note: If there's no leader, use velocity control
  xf : Inport
  vf : Inport  Port=2
  xl : Inport  Port=3
  vl : Inport  Port=4
  Anti-windup gain : Gain  Gain=sqrt(Ki/Kd)
  Gain3 : Gain  Gain=velFilterGain
  Headway error : Subsystem  mask{vLen=vLen, g0=g0, h=h}
      mask prompts: vLen "Vehicle Length"; g0 "Standstill Gap"; h "Time Headway"
      mask init:
      | vLen >= 0;
      | g0 >= 0;
      | h >= 0;
  Integrator : Integrator
  Integrator1 : Integrator  InitialCondition=initVel
  Integrator2 : Integrator
  Kd : Gain  Gain=Kd
  Ki : Gain  Gain=Ki
  Kp : Gain  Gain=Kp
  Mux : Mux  Inputs=2
  Rate Limiter : RateLimiter  RisingSlewLimit=maxJerk  FallingSlewLimit=minJerk  SampleTimeMode=inherited
  Saturation : Saturate  UpperLimit=maxAcceleration  LowerLimit=minAcceleration
  Saturation1 : Saturate  UpperLimit=maxHeadwayError  LowerLimit=minHeadwayError
  Saturation2 : Saturate  UpperLimit=maxAcc  LowerLimit=minAcc
  Sum : Sum  Inputs=-+
  Sum1 : Sum  Inputs=+++
  Sum2 : Sum  Inputs=|+-
  Sum3 : Sum
  Sum4 : Sum  Inputs=-+
  Sum5 : Sum  Inputs=++|
  Switch : Switch  Criteria=u2 > Threshold
  VelKi : Gain  Gain=VelKi
  u : Outport
  errors : Outport  Port=2
  gap : Outport  Port=3
  wires:
  Headway error/1(eh) -> Saturation1/1
  vf/1 -> Sum/1, Headway error/2(vf)
  Kd/1 -> Sum3/1, Sum1/3
  Kp/1 -> Sum1/2
  xl/1 -> Switch/2, Headway error/3(xl)
  xf/1 -> Headway error/1(xf)
  Gain3/1 -> Saturation/1
  Saturation/1 -> Integrator1/1
  Integrator1/1 -> Sum2/2, Sum/2
  vl/1 -> Sum2/1
  Sum2/1 -> Gain3/1
  Saturation1/1 -> Ki/1, Mux/1, Kp/1
  Headway error/2("gap ") -> gap/1
  Integrator2/1 -> VelKi/1
  VelKi/1 -> Sum3/2
  Switch/1 -> Sum4/1, Saturation2/1  "u"
  Sum1/1 -> Switch/1
  Sum3/1 -> Switch/3
  Sum/1 -> Integrator2/1, Mux/2, Kd/1
  Mux/1 -> errors/1
  Saturation2/1 -> Rate Limiter/1
  Integrator/1 -> Sum1/1
  Sum4/1 -> Anti-windup gain/1
  Ki/1 -> Sum5/2
  Sum5/1 -> Integrator/1
  Anti-windup gain/1 -> Sum5/1
  Rate Limiter/1 -> u/1, Sum4/2  "sat(u)"

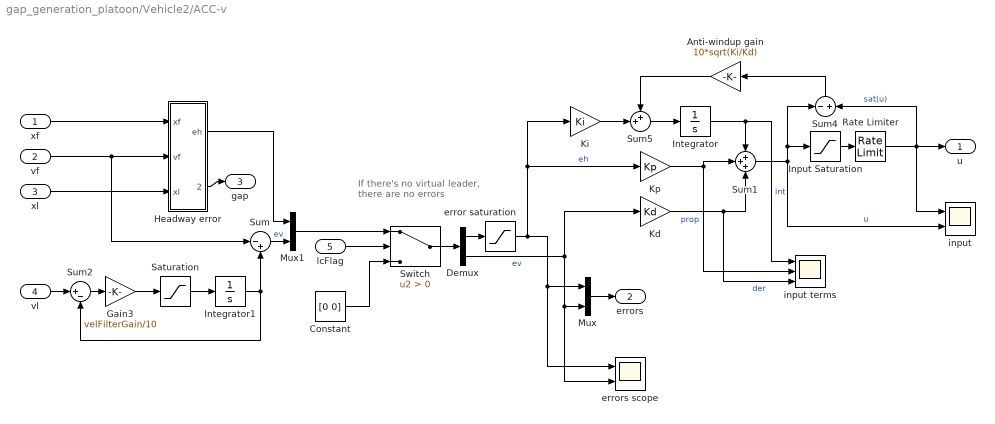
== system gap_generation_platoon/Vehicle2/ACC-v ==
  note: If there's no virtual leader,
      | there are no errors
  xf : Inport
  vf : Inport  Port=2
  xl : Inport  Port=3
  vl : Inport  Port=4
  lcFlag : Inport  Port=5
  Anti-windup gain : Gain  Gain=10*sqrt(Ki/Kd)
  Constant : Constant  Value=[0 0]
  Demux : Demux  Outputs=2
  Gain3 : Gain  Gain=velFilterGain/10
  Headway error : Subsystem  mask{vLen=vLen, g0=g0, h=h}
      mask prompts: vLen "Vehicle Length"; g0 "Standstill Gap"; h "Time Headway"
      mask init:
      | vLen >= 0;
      | g0 >= 0;
      | h >= 0;
  Input Saturation : Saturate  UpperLimit=maxAcc  LowerLimit=minAcc/4
  Integrator : Integrator
  Integrator1 : Integrator  InitialCondition=initVel
  Kd : Gain  Gain=Kd
  Ki : Gain  Gain=Ki
  Kp : Gain  Gain=Kp
  Mux : Mux  Inputs=2
  Mux1 : Mux  Inputs=2
  Rate Limiter : RateLimiter  RisingSlewLimit=maxJerk/2  FallingSlewLimit=minJerk/3  SampleTimeMode=inherited
  Saturation : Saturate  UpperLimit=maxAcceleration  LowerLimit=minAcceleration
  Sum : Sum  Inputs=|-+
  Sum1 : Sum  Inputs=+++
  Sum2 : Sum  Inputs=|+-
  Sum4 : Sum  Inputs=-+
  Sum5 : Sum  Inputs=++|
  Switch : Switch  Criteria=u2 > Threshold
  error saturation : Saturate  UpperLimit=maxHeadwayError  LowerLimit=minHeadwayError/10
  errors scope : Scope  NumInputPorts=2
  input : Scope  NumInputPorts=2
  input terms : Scope  NumInputPorts=3
  u : Outport
  errors : Outport  Port=2
  gap : Outport  Port=3
  wires:
  Headway error/1(eh) -> Mux1/1
  vf/1 -> Sum/1, Headway error/2(vf)
  Kd/1 -> input terms/3, Sum1/3  "der"
  Kp/1 -> input terms/2, Sum1/2  "prop"
  xf/1 -> Headway error/1(xf)
  Gain3/1 -> Saturation/1
  Saturation/1 -> Integrator1/1
  Integrator1/1 -> Sum2/2, Sum/2
  vl/1 -> Sum2/1
  Sum2/1 -> Gain3/1
  error saturation/1 -> Kp/1, Ki/1, errors scope/1, Mux/1  "eh"
  Headway error/2("gap ") -> gap/1
  xl/1 -> Headway error/3(xl)
  Sum1/1 -> input/2, Sum4/1, Input Saturation/1  "u"
  Sum/1 -> Mux1/2  "ev"
  Mux/1 -> errors/1
  Input Saturation/1 -> Rate Limiter/1
  Integrator/1 -> input terms/1, Sum1/1  "int"
  Sum4/1 -> Anti-windup gain/1
  Ki/1 -> Sum5/2
  Sum5/1 -> Integrator/1
  Anti-windup gain/1 -> Sum5/1
  Demux/2 -> Kd/1, errors scope/2, Mux/2  "ev"
  Demux/1 -> error saturation/1
  Switch/1 -> Demux/1
  Mux1/1 -> Switch/1
  lcFlag/1 -> Switch/2
  Constant/1 -> Switch/3
  Rate Limiter/1 -> input/1, u/1, Sum4/2  "sat(u)"

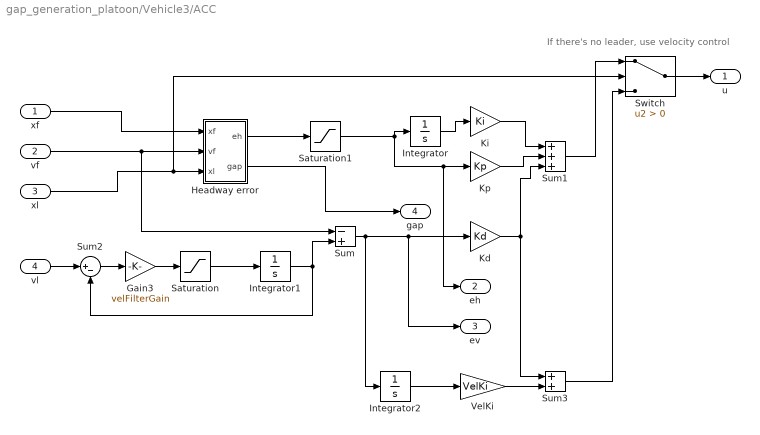
== system gap_generation_platoon/Vehicle3/ACC ==
  note: If there's no leader, use velocity control
  xf : Inport
  vf : Inport  Port=2
  xl : Inport  Port=3
  vl : Inport  Port=4
  Gain3 : Gain  Gain=velFilterGain
  Headway error : Subsystem  mask{vLen=vLen, g0=g0, h=h}
      mask prompts: vLen "Vehicle Length"; g0 "Standstill Gap"; h "Time Headway"
      mask init:
      | vLen >= 0;
      | g0 >= 0;
      | h >= 0;
  Integrator : Integrator
  Integrator1 : Integrator  InitialCondition=initVel
  Integrator2 : Integrator
  Kd : Gain  Gain=Kd
  Ki : Gain  Gain=Ki
  Kp : Gain  Gain=Kp
  Saturation : Saturate  UpperLimit=maxAcceleration  LowerLimit=minAcceleration
  Saturation1 : Saturate  UpperLimit=maxHeadwayError  LowerLimit=minHeadwayError
  Sum : Sum  Inputs=-+
  Sum1 : Sum  Inputs=+++
  Sum2 : Sum  Inputs=|+-
  Sum3 : Sum
  Switch : Switch  Criteria=u2 > Threshold
  VelKi : Gain  Gain=VelKi
  u : Outport
  eh : Outport  Port=2
  ev : Outport  Port=3
  gap : Outport  Port=4
  wires:
  Headway error/1(eh) -> Saturation1/1
  vf/1 -> Sum/1, Headway error/2(vf)
  Kd/1 -> Sum3/1, Sum1/3
  Kp/1 -> Sum1/2
  Ki/1 -> Sum1/1
  Integrator/1 -> Ki/1
  xl/1 -> Switch/2, Headway error/3(xl)
  xf/1 -> Headway error/1(xf)
  Gain3/1 -> Saturation/1
  Saturation/1 -> Integrator1/1
  Integrator1/1 -> Sum2/2, Sum/2
  vl/1 -> Sum2/1
  Sum2/1 -> Gain3/1
  Saturation1/1 -> eh/1, Kp/1, Integrator/1
  Headway error/2("gap ") -> gap/1
  Integrator2/1 -> VelKi/1
  VelKi/1 -> Sum3/2
  Switch/1 -> u/1
  Sum1/1 -> Switch/1
  Sum3/1 -> Switch/3
  Sum/1 -> Integrator2/1, ev/1, Kd/1

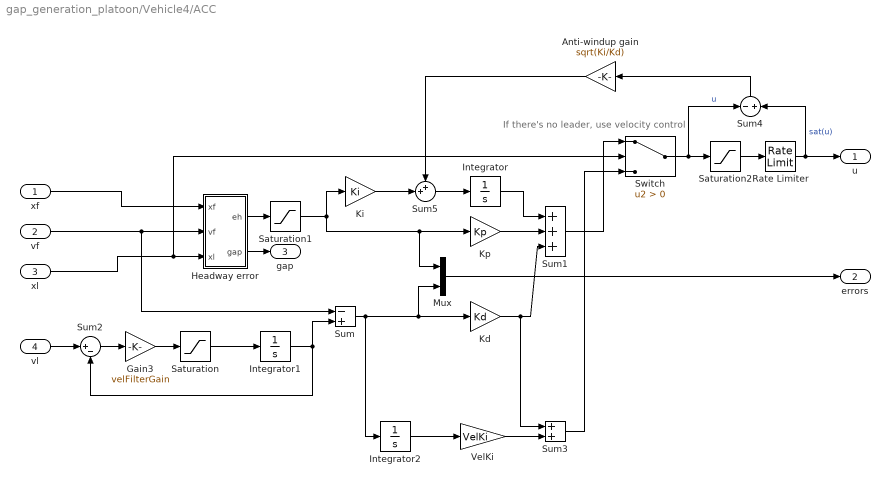
== system gap_generation_platoon/Vehicle4/ACC ==
  note: If there's no leader, use velocity control
  xf : Inport
  vf : Inport  Port=2
  xl : Inport  Port=3
  vl : Inport  Port=4
  Anti-windup gain : Gain  Gain=sqrt(Ki/Kd)
  Gain3 : Gain  Gain=velFilterGain
  Headway error : Subsystem  mask{vLen=vLen, g0=g0, h=h}
      mask prompts: vLen "Vehicle Length"; g0 "Standstill Gap"; h "Time Headway"
      mask init:
      | vLen >= 0;
      | g0 >= 0;
      | h >= 0;
  Integrator : Integrator
  Integrator1 : Integrator  InitialCondition=initVel
  Integrator2 : Integrator
  Kd : Gain  Gain=Kd
  Ki : Gain  Gain=Ki
  Kp : Gain  Gain=Kp
  Mux : Mux  Inputs=2
  Rate Limiter : RateLimiter  RisingSlewLimit=maxJerk  FallingSlewLimit=minJerk  SampleTimeMode=inherited
  Saturation : Saturate  UpperLimit=maxAcceleration  LowerLimit=minAcceleration
  Saturation1 : Saturate  UpperLimit=maxHeadwayError  LowerLimit=minHeadwayError
  Saturation2 : Saturate  UpperLimit=maxAcc  LowerLimit=minAcc
  Sum : Sum  Inputs=-+
  Sum1 : Sum  Inputs=+++
  Sum2 : Sum  Inputs=|+-
  Sum3 : Sum
  Sum4 : Sum  Inputs=-+
  Sum5 : Sum  Inputs=++|
  Switch : Switch  Criteria=u2 > Threshold
  VelKi : Gain  Gain=VelKi
  u : Outport
  errors : Outport  Port=2
  gap : Outport  Port=3
  wires:
  Headway error/1(eh) -> Saturation1/1
  vf/1 -> Sum/1, Headway error/2(vf)
  Kd/1 -> Sum3/1, Sum1/3
  Kp/1 -> Sum1/2
  xl/1 -> Switch/2, Headway error/3(xl)
  xf/1 -> Headway error/1(xf)
  Gain3/1 -> Saturation/1
  Saturation/1 -> Integrator1/1
  Integrator1/1 -> Sum2/2, Sum/2
  vl/1 -> Sum2/1
  Sum2/1 -> Gain3/1
  Saturation1/1 -> Ki/1, Mux/1, Kp/1
  Headway error/2("gap ") -> gap/1
  Integrator2/1 -> VelKi/1
  VelKi/1 -> Sum3/2
  Switch/1 -> Sum4/1, Saturation2/1  "u"
  Sum1/1 -> Switch/1
  Sum3/1 -> Switch/3
  Sum/1 -> Integrator2/1, Mux/2, Kd/1
  Mux/1 -> errors/1
  Saturation2/1 -> Rate Limiter/1
  Integrator/1 -> Sum1/1
  Sum4/1 -> Anti-windup gain/1
  Ki/1 -> Sum5/2
  Sum5/1 -> Integrator/1
  Anti-windup gain/1 -> Sum5/1
  Rate Limiter/1 -> u/1, Sum4/2  "sat(u)"

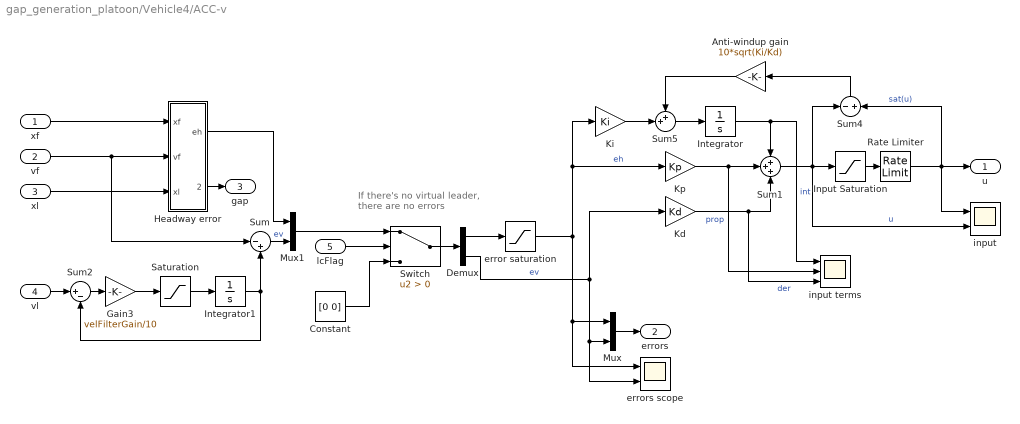
== system gap_generation_platoon/Vehicle4/ACC-v ==
  note: If there's no virtual leader,
      | there are no errors
  xf : Inport
  vf : Inport  Port=2
  xl : Inport  Port=3
  vl : Inport  Port=4
  lcFlag : Inport  Port=5
  Anti-windup gain : Gain  Gain=10*sqrt(Ki/Kd)
  Constant : Constant  Value=[0 0]
  Demux : Demux  Outputs=2
  Gain3 : Gain  Gain=velFilterGain/10
  Headway error : Subsystem  mask{vLen=vLen, g0=g0, h=h}
      mask prompts: vLen "Vehicle Length"; g0 "Standstill Gap"; h "Time Headway"
      mask init:
      | vLen >= 0;
      | g0 >= 0;
      | h >= 0;
  Input Saturation : Saturate  UpperLimit=maxAcc  LowerLimit=minAcc/4
  Integrator : Integrator
  Integrator1 : Integrator  InitialCondition=initVel
  Kd : Gain  Gain=Kd
  Ki : Gain  Gain=Ki
  Kp : Gain  Gain=Kp
  Mux : Mux  Inputs=2
  Mux1 : Mux  Inputs=2
  Rate Limiter : RateLimiter  RisingSlewLimit=maxJerk/2  FallingSlewLimit=minJerk/3  SampleTimeMode=inherited
  Saturation : Saturate  UpperLimit=maxAcceleration  LowerLimit=minAcceleration
  Sum : Sum  Inputs=|-+
  Sum1 : Sum  Inputs=+++
  Sum2 : Sum  Inputs=|+-
  Sum4 : Sum  Inputs=-+
  Sum5 : Sum  Inputs=++|
  Switch : Switch  Criteria=u2 > Threshold
  error saturation : Saturate  UpperLimit=maxHeadwayError  LowerLimit=minHeadwayError/10
  errors scope : Scope  NumInputPorts=2
  input : Scope  NumInputPorts=2
  input terms : Scope  NumInputPorts=3
  u : Outport
  errors : Outport  Port=2
  gap : Outport  Port=3
  wires:
  Headway error/1(eh) -> Mux1/1
  vf/1 -> Sum/1, Headway error/2(vf)
  Kd/1 -> input terms/3, Sum1/3  "der"
  Kp/1 -> input terms/2, Sum1/2  "prop"
  xf/1 -> Headway error/1(xf)
  Gain3/1 -> Saturation/1
  Saturation/1 -> Integrator1/1
  Integrator1/1 -> Sum2/2, Sum/2
  vl/1 -> Sum2/1
  Sum2/1 -> Gain3/1
  error saturation/1 -> Kp/1, Ki/1, errors scope/1, Mux/1  "eh"
  Headway error/2("gap ") -> gap/1
  xl/1 -> Headway error/3(xl)
  Sum1/1 -> Sum4/1, Input Saturation/1, input/2  "u"
  Sum/1 -> Mux1/2  "ev"
  Mux/1 -> errors/1
  Input Saturation/1 -> Rate Limiter/1
  Integrator/1 -> input terms/1, Sum1/1  "int"
  Sum4/1 -> Anti-windup gain/1
  Ki/1 -> Sum5/2
  Sum5/1 -> Integrator/1
  Anti-windup gain/1 -> Sum5/1
  Demux/2 -> Kd/1, errors scope/2, Mux/2  "ev"
  Demux/1 -> error saturation/1
  Switch/1 -> Demux/1
  Mux1/1 -> Switch/1
  lcFlag/1 -> Switch/2
  Constant/1 -> Switch/3
  Rate Limiter/1 -> Sum4/2, u/1, input/1  "sat(u)"

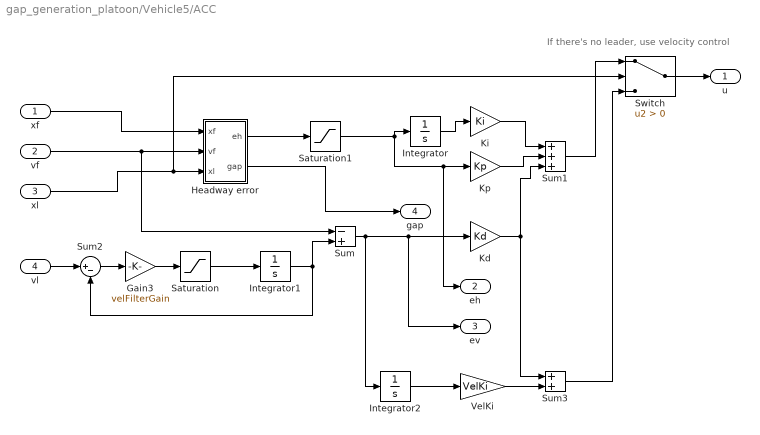
== system gap_generation_platoon/Vehicle5/ACC ==
  note: If there's no leader, use velocity control
  xf : Inport
  vf : Inport  Port=2
  xl : Inport  Port=3
  vl : Inport  Port=4
  Gain3 : Gain  Gain=velFilterGain
  Headway error : Subsystem  mask{vLen=vLen, g0=g0, h=h}
      mask prompts: vLen "Vehicle Length"; g0 "Standstill Gap"; h "Time Headway"
      mask init:
      | vLen >= 0;
      | g0 >= 0;
      | h >= 0;
  Integrator : Integrator
  Integrator1 : Integrator  InitialCondition=initVel
  Integrator2 : Integrator
  Kd : Gain  Gain=Kd
  Ki : Gain  Gain=Ki
  Kp : Gain  Gain=Kp
  Saturation : Saturate  UpperLimit=maxAcceleration  LowerLimit=minAcceleration
  Saturation1 : Saturate  UpperLimit=maxHeadwayError  LowerLimit=minHeadwayError
  Sum : Sum  Inputs=-+
  Sum1 : Sum  Inputs=+++
  Sum2 : Sum  Inputs=|+-
  Sum3 : Sum
  Switch : Switch  Criteria=u2 > Threshold
  VelKi : Gain  Gain=VelKi
  u : Outport
  eh : Outport  Port=2
  ev : Outport  Port=3
  gap : Outport  Port=4
  wires:
  Headway error/1(eh) -> Saturation1/1
  vf/1 -> Sum/1, Headway error/2(vf)
  Kd/1 -> Sum3/1, Sum1/3
  Kp/1 -> Sum1/2
  Ki/1 -> Sum1/1
  Integrator/1 -> Ki/1
  xl/1 -> Switch/2, Headway error/3(xl)
  xf/1 -> Headway error/1(xf)
  Gain3/1 -> Saturation/1
  Saturation/1 -> Integrator1/1
  Integrator1/1 -> Sum2/2, Sum/2
  vl/1 -> Sum2/1
  Sum2/1 -> Gain3/1
  Saturation1/1 -> eh/1, Kp/1, Integrator/1
  Headway error/2("gap ") -> gap/1
  Integrator2/1 -> VelKi/1
  VelKi/1 -> Sum3/2
  Switch/1 -> u/1
  Sum1/1 -> Switch/1
  Sum3/1 -> Switch/3
  Sum/1 -> Integrator2/1, ev/1, Kd/1

== system gap_generation_platoon/Vehicle1/ACC/Headway error ==
  note: gap
  note: x (front bumper)
  xf : Inport
  vf : Inport  Port=2
  xl : Inport  Port=3
  Multiply : Product
  Sum : Sum  Inputs=-+
  Sum1 : Sum
  Sum2 : Sum  Inputs=+-|
  Sum3 : Sum  Inputs=+-
  g0 : Constant  Value=g0
  h : Constant  Value=h
  vLen : Constant  Value=vLen
  eh : Outport
  "gap " : Outport  Port=2
  wires:
  vLen/1 -> Sum1/1
  Multiply/1 -> Sum3/2
  g0/1 -> Sum2/2
  Sum2/1 -> Sum3/1
  Sum/1 -> "gap "/1, Sum2/1
  xf/1 -> Sum1/2
  Sum3/1 -> eh/1
  vf/1 -> Multiply/1
  h/1 -> Multiply/2
  Sum1/1 -> Sum/1
  xl/1 -> Sum/2

== system gap_generation_platoon/Vehicle2/ACC/Headway error ==
  note: gap
  note: x (front bumper)
  xf : Inport
  vf : Inport  Port=2
  xl : Inport  Port=3
  Multiply : Product
  Sum : Sum  Inputs=-+
  Sum1 : Sum
  Sum2 : Sum  Inputs=+-|
  Sum3 : Sum  Inputs=+-
  g0 : Constant  Value=g0
  h : Constant  Value=h
  vLen : Constant  Value=vLen
  eh : Outport
  "gap " : Outport  Port=2
  wires:
  vLen/1 -> Sum1/1
  Multiply/1 -> Sum3/2
  g0/1 -> Sum2/2
  Sum2/1 -> Sum3/1
  Sum/1 -> "gap "/1, Sum2/1
  xf/1 -> Sum1/2
  Sum3/1 -> eh/1
  vf/1 -> Multiply/1
  h/1 -> Multiply/2
  Sum1/1 -> Sum/1
  xl/1 -> Sum/2

== system gap_generation_platoon/Vehicle2/ACC-v/Headway error ==
  note: gap
  note: x (front bumper)
  xf : Inport
  vf : Inport  Port=2
  xl : Inport  Port=3
  Multiply : Product
  Sum : Sum  Inputs=-+
  Sum1 : Sum
  Sum2 : Sum  Inputs=+-|
  Sum3 : Sum  Inputs=+-
  g0 : Constant  Value=g0
  h : Constant  Value=h
  vLen : Constant  Value=vLen
  eh : Outport
  "gap " : Outport  Port=2
  wires:
  vLen/1 -> Sum1/1
  Multiply/1 -> Sum3/2
  g0/1 -> Sum2/2
  Sum2/1 -> Sum3/1
  Sum/1 -> "gap "/1, Sum2/1
  xf/1 -> Sum1/2
  Sum3/1 -> eh/1
  vf/1 -> Multiply/1
  h/1 -> Multiply/2
  Sum1/1 -> Sum/1
  xl/1 -> Sum/2

== system gap_generation_platoon/Vehicle3/ACC/Headway error ==
  note: gap
  note: x (front bumper)
  xf : Inport
  vf : Inport  Port=2
  xl : Inport  Port=3
  Multiply : Product
  Sum : Sum  Inputs=-+
  Sum1 : Sum
  Sum2 : Sum  Inputs=+-|
  Sum3 : Sum  Inputs=+-
  g0 : Constant  Value=g0
  h : Constant  Value=h
  vLen : Constant  Value=vLen
  eh : Outport
  "gap " : Outport  Port=2
  wires:
  vLen/1 -> Sum1/1
  Multiply/1 -> Sum3/2
  g0/1 -> Sum2/2
  Sum2/1 -> Sum3/1
  Sum/1 -> "gap "/1, Sum2/1
  xf/1 -> Sum1/2
  Sum3/1 -> eh/1
  vf/1 -> Multiply/1
  h/1 -> Multiply/2
  Sum1/1 -> Sum/1
  xl/1 -> Sum/2

== system gap_generation_platoon/Vehicle4/ACC/Headway error ==
  note: gap
  note: x (front bumper)
  xf : Inport
  vf : Inport  Port=2
  xl : Inport  Port=3
  Multiply : Product
  Sum : Sum  Inputs=-+
  Sum1 : Sum
  Sum2 : Sum  Inputs=+-|
  Sum3 : Sum  Inputs=+-
  g0 : Constant  Value=g0
  h : Constant  Value=h
  vLen : Constant  Value=vLen
  eh : Outport
  "gap " : Outport  Port=2
  wires:
  vLen/1 -> Sum1/1
  Multiply/1 -> Sum3/2
  g0/1 -> Sum2/2
  Sum2/1 -> Sum3/1
  Sum/1 -> "gap "/1, Sum2/1
  xf/1 -> Sum1/2
  Sum3/1 -> eh/1
  vf/1 -> Multiply/1
  h/1 -> Multiply/2
  Sum1/1 -> Sum/1
  xl/1 -> Sum/2

== system gap_generation_platoon/Vehicle4/ACC-v/Headway error ==
  note: gap
  note: x (front bumper)
  xf : Inport
  vf : Inport  Port=2
  xl : Inport  Port=3
  Multiply : Product
  Sum : Sum  Inputs=-+
  Sum1 : Sum
  Sum2 : Sum  Inputs=+-|
  Sum3 : Sum  Inputs=+-
  g0 : Constant  Value=g0
  h : Constant  Value=h
  vLen : Constant  Value=vLen
  eh : Outport
  "gap " : Outport  Port=2
  wires:
  vLen/1 -> Sum1/1
  Multiply/1 -> Sum3/2
  g0/1 -> Sum2/2
  Sum2/1 -> Sum3/1
  Sum/1 -> "gap "/1, Sum2/1
  xf/1 -> Sum1/2
  Sum3/1 -> eh/1
  vf/1 -> Multiply/1
  h/1 -> Multiply/2
  Sum1/1 -> Sum/1
  xl/1 -> Sum/2

== system gap_generation_platoon/Vehicle5/ACC/Headway error ==
  note: gap
  note: x (front bumper)
  xf : Inport
  vf : Inport  Port=2
  xl : Inport  Port=3
  Multiply : Product
  Sum : Sum  Inputs=-+
  Sum1 : Sum
  Sum2 : Sum  Inputs=+-|
  Sum3 : Sum  Inputs=+-
  g0 : Constant  Value=g0
  h : Constant  Value=h
  vLen : Constant  Value=vLen
  eh : Outport
  "gap " : Outport  Port=2
  wires:
  vLen/1 -> Sum1/1
  Multiply/1 -> Sum3/2
  g0/1 -> Sum2/2
  Sum2/1 -> Sum3/1
  Sum/1 -> "gap "/1, Sum2/1
  xf/1 -> Sum1/2
  Sum3/1 -> eh/1
  vf/1 -> Multiply/1
  h/1 -> Multiply/2
  Sum1/1 -> Sum/1
  xl/1 -> Sum/2
